simulink model "three_phase_inverter"  (R2024b)
settings: Solver=VariableStepAuto  StartTime=0.0  StopTime=1  RelTol=1e-3
libraries: spsIGBTLib x6, spsVoltageMeasurementLib x6, spsCurrentMeasurementLib x3, spsSeriesRLCBranchLib x3, spsDCVoltageSourceLib x1, simulink x1, sps_lib x1
settings Model: Creator=sanja  LastModifiedBy=sanja

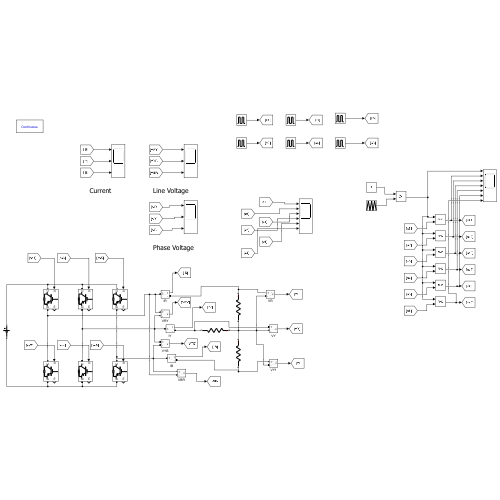
[thumbnail: Simulink's stored preview of the top-level diagram]
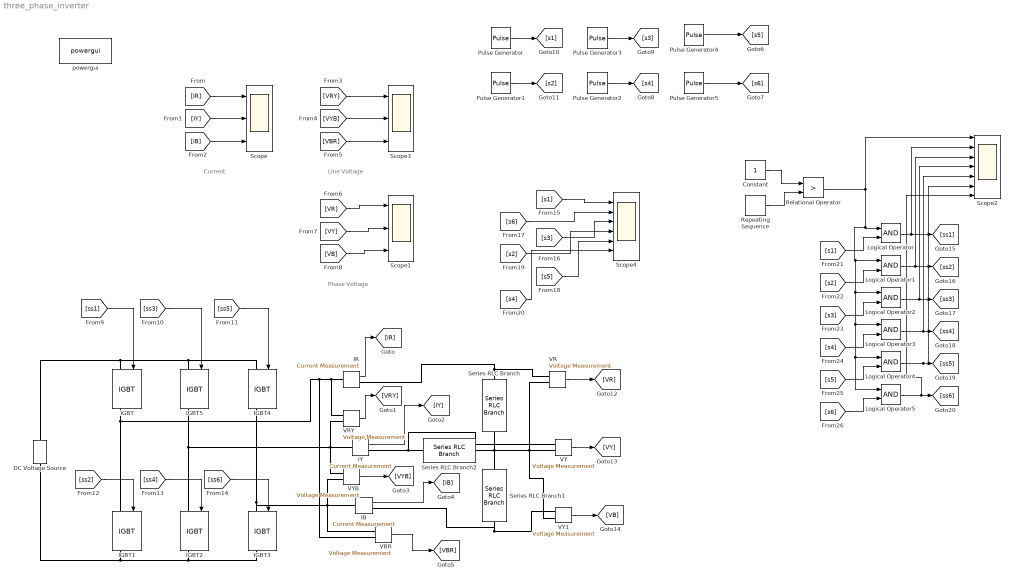
== system three_phase_inverter ==
  note: Current
  note: Line Voltage
  note: Phase Voltage
  Constant : Constant
  DC Voltage Source : spsDCVoltageSourceLib/DC Voltage Source  Amplitude=100  Measurements=None
  IB : spsCurrentMeasurementLib/Current Measurement  PhasorSimulation=off  OutputType=Complex  PSBequivalent=0
  IGBT{,1..5} (6 alike) : spsIGBTLib/IGBT  Ron=0.001  Lon=0  Vf=1  Tf=1e-6  Tt=2e-6  IC=0  Rs=1e5  Cs=inf  Measurements=on
  IR : spsCurrentMeasurementLib/Current Measurement  PhasorSimulation=off  OutputType=Complex  PSBequivalent=0
  IY : spsCurrentMeasurementLib/Current Measurement  PhasorSimulation=off  OutputType=Complex  PSBequivalent=0
  Logical Operator{,1..5} (6 alike) : Logic  AllPortsSameDT=off  OutDataTypeStr=boolean
  Pulse Generator : DiscretePulseGenerator  PulseType=Time based  Period=0.02  PulseWidth=50
  Pulse Generator1 : DiscretePulseGenerator  PulseType=Time based  Period=0.02  PulseWidth=50  PhaseDelay=180*0.02/360
  Pulse Generator2 : DiscretePulseGenerator  PulseType=Time based  Period=0.02  PulseWidth=50  PhaseDelay=300*0.02/360
  Pulse Generator3 : DiscretePulseGenerator  PulseType=Time based  Period=0.02  PulseWidth=50  PhaseDelay=120*0.02/360
  Pulse Generator4 : DiscretePulseGenerator  PulseType=Time based  Period=0.02  PulseWidth=50  PhaseDelay=240*0.02/360
  Pulse Generator5 : DiscretePulseGenerator  PulseType=Time based  Period=0.02  PulseWidth=50  PhaseDelay=60*0.02/360
  Relational Operator : RelationalOperator  Operator=>  OutDataTypeStr=boolean  RndMeth=Simplest  InputSameDT=off
  Repeating Sequence : simulink/Sources/Repeating Sequence  rep_seq_t=[0 0.02/40 0.02/20]  rep_seq_y=[0 2 0]
  Scope : Scope  NumInputPorts=3
  Scope1 : Scope  NumInputPorts=3
  Scope2 : Scope  NumInputPorts=7
  Scope3 : Scope  NumInputPorts=3
  Scope4 : Scope  NumInputPorts=6
  Series RLC Branch : spsSeriesRLCBranchLib/Series RLC Branch  LConnTagsString=__new0  RConnTagsString=__new0  BranchType=R  Resistance=1  Inductance=1e-3  SetiL0=off  InitialCurrent=0  Capacitance=1e-6  Setx0=off  InitialVoltage=0  Measurements=None
  Series RLC Branch1 : spsSeriesRLCBranchLib/Series RLC Branch  LConnTagsString=__new0  RConnTagsString=__new0  BranchType=R  Resistance=1  Inductance=1e-3  SetiL0=off  InitialCurrent=0  Capacitance=1e-6  Setx0=off  InitialVoltage=0  Measurements=None
  Series RLC Branch2 : spsSeriesRLCBranchLib/Series RLC Branch  LConnTagsString=__new0  RConnTagsString=__new0  BranchType=R  Resistance=1  Inductance=1e-3  SetiL0=off  InitialCurrent=0  Capacitance=1e-6  Setx0=off  InitialVoltage=0  Measurements=None
  VBR : spsVoltageMeasurementLib/Voltage Measurement  PhasorSimulation=off  OutputType=Complex  PSBequivalent=0
  VR : spsVoltageMeasurementLib/Voltage Measurement  PhasorSimulation=off  OutputType=Complex  PSBequivalent=0
  VRY : spsVoltageMeasurementLib/Voltage Measurement  PhasorSimulation=off  OutputType=Complex  PSBequivalent=0
  VY : spsVoltageMeasurementLib/Voltage Measurement  PhasorSimulation=off  OutputType=Complex  PSBequivalent=0
  VY1 : spsVoltageMeasurementLib/Voltage Measurement  PhasorSimulation=off  OutputType=Complex  PSBequivalent=0
  VYB : spsVoltageMeasurementLib/Voltage Measurement  PhasorSimulation=off  OutputType=Complex  PSBequivalent=0
  powergui : sps_lib/powergui  Priority=1  SimulationMode=Continuous  SampleTime=50e-6  frequency=60  Iterations=50  frequencyindice=0  Pbase=100e6  ErrMax=1e-4  UnitsV=kV  UnitsW=MW  buscounter=0  FunctionMessages=off  echomessages=off  EnableUseOfTLC=off  CurrentSourceSwitches=off  DisableSnubberDevices=off  DisableRonSwitches=off  DisableVfSwitches=off  DisplayEquations=off  AutomaticDiscreteSolvers=off  SolverType=Tustin/Backward Euler (TBE)  Interpol=off  ExternalGateDelay=off  methode=off  Ts=100  x0status=blocks  SPID=on  SwTol=0  HookPort=off  NonlinearTolerance=1e-4  nMaxIteration=100  ContinueOnMaxIteration=off  RestoreLinks=warning  ResistiveCurrentMeasurement=off  Frange=[0:2:500]  Ylog=off  Xlog=on  ShowGrid=off  save=off  variable=ZData  structure=0  ZoomFFT=off  StartTime=0.0  cycles=1  DisplayStyle=1  fundamental=60  FreqAxis=off  MaxFrequency=1000  frequencyindicesteady=1  RmsSteady=1  display=off
  wires:
  [IR] -> Scope/1
  [IY] -> Scope/2
  [IB] -> Scope/3
  [VRY] -> Scope3/1
  [VYB] -> Scope3/2
  [VBR] -> Scope3/3
  [VR] -> Scope1/1
  [VY] -> Scope1/2
  [VB] -> Scope1/3
  IR/1 -> [IR]
  VRY/1 -> [VRY]
  IY/1 -> [IY]
  VYB/1 -> [VYB]
  IB/1 -> [IB]
  VBR/1 -> [VBR]
  Pulse Generator/1 -> [s1]
  Pulse Generator1/1 -> [s2]
  Pulse Generator3/1 -> [s3]
  Pulse Generator2/1 -> [s4]
  Pulse Generator4/1 -> [s5]
  Pulse Generator5/1 -> [s6]
  [ss1] -> IGBT/1
  [ss3] -> IGBT5/1
  [ss5] -> IGBT4/1
  [ss2] -> IGBT1/1
  [ss4] -> IGBT2/1
  [ss6] -> IGBT3/1
  [s1] -> Scope4/1
  [s6] -> Scope4/2
  [s3] -> Scope4/3
  [s2] -> Scope4/4
  [s5] -> Scope4/5
  [s4] -> Scope4/6
  VY/1 -> [VY]
  VR/1 -> [VR]
  VY1/1 -> [VB]
  Relational Operator/1 -> Scope2/1, Logical Operator5/1, Logical Operator4/1, Logical Operator3/1, Logical Operator2/1, Logical Operator1/1, Logical Operator/1
  Constant/1 -> Relational Operator/1
  Repeating Sequence/1 -> Relational Operator/2
  [s1] -> Logical Operator/2
  [s2] -> Logical Operator1/2
  [s3] -> Logical Operator2/2
  [s4] -> Logical Operator3/2
  [s5] -> Logical Operator4/2
  [s6] -> Logical Operator5/2
  Logical Operator/1 -> Scope2/2, [ss1]
  Logical Operator1/1 -> Scope2/3, [ss2]
  Logical Operator2/1 -> Scope2/4, [ss3]
  Logical Operator3/1 -> Scope2/5, [ss4]
  Logical Operator4/1 -> Scope2/6, [ss5]
  Logical Operator5/1 -> Scope2/7, [ss6]
  connections:
  IGBT/RConn1 -- VBR/LConn2 -- VRY/LConn1 -- IR/LConn1 -- IGBT1/LConn1
  IGBT5/RConn1 -- IGBT2/LConn1 -- VRY/LConn2 -- VYB/LConn1 -- IY/LConn1
  IGBT4/RConn1 -- VYB/LConn2 -- VBR/LConn1 -- IB/LConn1 -- IGBT3/LConn1
  IGBT/LConn1 -- IGBT5/LConn1 -- IGBT4/LConn1 -- DC Voltage Source/RConn1
  IGBT1/RConn1 -- IGBT2/RConn1 -- IGBT3/RConn1 -- DC Voltage Source/LConn1
  VR/LConn2 -- Series RLC Branch2/LConn1 -- Series RLC Branch1/LConn1 -- Series RLC Branch/RConn1 -- VY1/LConn2 -- VY/LConn2
  IY/RConn1 -- VY/LConn1 -- Series RLC Branch2/RConn1
  IB/RConn1 -- VY1/LConn1 -- Series RLC Branch1/RConn1
  Series RLC Branch/LConn1 -- VR/LConn1 -- IR/RConn1
